simulink model "hw3_scattering_teleop_FP_nodamp"  (R2023b)
settings: Solver=ode45  StartTime=0.0  StopTime=10.0  FixedStep=0.001  RelTol=1e-3
values from neighbouring files (symbols this model uses):
  A = 1    [Copy_of_hw1_four_channel_bilateral_teleoperation_params.m]    (also in hw1_four_channel_bilateral_teleoperation_params.m; hw2_2_3_channel_bilateral_teleoperation_params.m; hw3_scattering_teleop_FP_params.m = 1.5; hw3_scattering_teleop_PP_params.m)
  Ak = [1 Ts ... (first row only)    [hw3_scattering_teleop_FP_params.m]    (also in hw3_scattering_teleop_PP_params.m; hw4_tank_FP_params.m; hw4_tank_PP_params.m; no_noise_hw4_tank_PP_params.m)
  B = [Ts^2/2; Ts]    [hw3_scattering_teleop_FP_params.m]    (also in hw3_scattering_teleop_PP_params.m; hw4_tank_FP_params.m; hw4_tank_PP_params.m; no_noise_hw4_tank_PP_params.m)
  b = 1    [hw3_scattering_teleop_FP_params.m]    (also in hw3_scattering_teleop_PP_params.m)
  Be = 100    [Copy_of_hw1_four_channel_bilateral_teleoperation_params.m]    (also in hw1_four_channel_bilateral_teleoperation_params.m; hw2_2_3_channel_bilateral_teleoperation_params.m; hw3_scattering_teleop_FP_params.m; hw3_scattering_teleop_PP_params.m)
  Bh = 1    [Copy_of_hw1_four_channel_bilateral_teleoperation_params.m]    (also in hw1_four_channel_bilateral_teleoperation_params.m; hw2_2_3_channel_bilateral_teleoperation_params.m; hw3_scattering_teleop_FP_params.m; hw3_scattering_teleop_PP_params.m)
  Bs = 4*Bm    (= 64)    [Copy_of_hw1_four_channel_bilateral_teleoperation_params.m]    (also in hw1_four_channel_bilateral_teleoperation_params.m; hw2_2_3_channel_bilateral_teleoperation_params.m; hw3_scattering_teleop_FP_params.m; hw3_scattering_teleop_PP_params.m)
  C = [1 0]    [hw3_scattering_teleop_FP_params.m]    (also in hw3_scattering_teleop_PP_params.m; hw4_tank_FP_params.m; hw4_tank_PP_params.m; no_noise_hw4_tank_PP_params.m)
  d = 1    [hw2_2_3_channel_bilateral_teleoperation_params.m]    (also in hw3_scattering_teleop_FP_params.m = 10; hw3_scattering_teleop_PP_params.m = 10; hw4_tank_FP_params.m = 10; hw4_tank_PP_params.m = 10)
  Dh = 20*0.8    (= 16)    [Copy_of_hw1_four_channel_bilateral_teleoperation_params.m]    (also in hw1_four_channel_bilateral_teleoperation_params.m; hw2_2_3_channel_bilateral_teleoperation_params.m; hw3_scattering_teleop_FP_params.m; hw3_scattering_teleop_PP_params.m)
  Dm = 5    [Copy_of_hw1_four_channel_bilateral_teleoperation_params.m]    (also in hw1_four_channel_bilateral_teleoperation_params.m; hw2_2_3_channel_bilateral_teleoperation_params.m; hw3_scattering_teleop_FP_params.m; hw3_scattering_teleop_PP_params.m = 0)
  Ds = 10    [Copy_of_hw1_four_channel_bilateral_teleoperation_params.m]    (also in hw1_four_channel_bilateral_teleoperation_params.m; hw2_2_3_channel_bilateral_teleoperation_params.m; hw3_scattering_teleop_FP_params.m = 0; hw3_scattering_teleop_PP_params.m = 0)
  Fc = 1    [Copy_of_hw1_four_channel_bilateral_teleoperation_params.m]    (also in hw1_four_channel_bilateral_teleoperation_params.m; hw2_2_3_channel_bilateral_teleoperation_params.m; hw3_scattering_teleop_FP_params.m; hw3_scattering_teleop_PP_params.m)
  Fip = 5    [hw3_scattering_teleop_FP_params.m]    (also in hw3_scattering_teleop_PP_params.m)
  Flp = 0.5    [Copy_of_hw1_four_channel_bilateral_teleoperation_params.m]    (also in hw1_four_channel_bilateral_teleoperation_params.m; hw2_2_3_channel_bilateral_teleoperation_params.m; hw3_scattering_teleop_FP_params.m = 0.01; hw3_scattering_teleop_PP_params.m = 0.01)
  Flp1 = 0.5    [hw3_scattering_teleop_FP_params.m]    (also in hw3_scattering_teleop_PP_params.m; hw4_tank_FP_params.m; hw4_tank_PP_params.m; no_noise_hw4_tank_PP_params.m)
  Jh = 1    [Copy_of_hw1_four_channel_bilateral_teleoperation_params.m]    (also in hw1_four_channel_bilateral_teleoperation_params.m; hw2_2_3_channel_bilateral_teleoperation_params.m; hw3_scattering_teleop_FP_params.m; hw3_scattering_teleop_PP_params.m)
  Ke = 200    [Copy_of_hw1_four_channel_bilateral_teleoperation_params.m]    (also in hw1_four_channel_bilateral_teleoperation_params.m; hw2_2_3_channel_bilateral_teleoperation_params.m; hw3_scattering_teleop_FP_params.m; hw3_scattering_teleop_PP_params.m)
  Kh = 0    [hw3_scattering_teleop_FP_params.m]    (also in hw3_scattering_teleop_PP_params.m; hw4_tank_FP_params.m; hw4_tank_PP_params.m; no_noise_hw4_tank_PP_params.m)
  Ks = 4*Km    (= 40)    [Copy_of_hw1_four_channel_bilateral_teleoperation_params.m]    (also in hw1_four_channel_bilateral_teleoperation_params.m; hw2_2_3_channel_bilateral_teleoperation_params.m; hw3_scattering_teleop_FP_params.m; hw3_scattering_teleop_PP_params.m)
  Mm = 0.5    [Copy_of_hw1_four_channel_bilateral_teleoperation_params.m]    (also in hw1_four_channel_bilateral_teleoperation_params.m; hw2_2_3_channel_bilateral_teleoperation_params.m; hw3_scattering_teleop_FP_params.m; hw3_scattering_teleop_PP_params.m)
  Ms = 2    [Copy_of_hw1_four_channel_bilateral_teleoperation_params.m]    (also in hw1_four_channel_bilateral_teleoperation_params.m; hw2_2_3_channel_bilateral_teleoperation_params.m; hw3_scattering_teleop_FP_params.m; hw3_scattering_teleop_PP_params.m)
  noise = 0.001    [hw3_scattering_teleop_FP_params.m]    (also in hw3_scattering_teleop_PP_params.m; hw4_tank_FP_params.m = 0.0001; hw4_tank_PP_params.m; no_noise_hw4_tank_PP_params.m)
  Ph = 10*1    (= 10)    [Copy_of_hw1_four_channel_bilateral_teleoperation_params.m]    (also in hw1_four_channel_bilateral_teleoperation_params.m; hw2_2_3_channel_bilateral_teleoperation_params.m; hw3_scattering_teleop_FP_params.m; hw3_scattering_teleop_PP_params.m)
  R = 1    [hw3_scattering_teleop_FP_params.m]    (also in hw3_scattering_teleop_PP_params.m; hw4_tank_FP_params.m; hw4_tank_PP_params.m; no_noise_hw4_tank_PP_params.m)
  Ts = 0.001    [hw3_scattering_teleop_FP_params.m]    (also in hw3_scattering_teleop_PP_params.m; hw4_tank_FP_params.m; hw4_tank_PP_params.m; no_noise_hw4_tank_PP_params.m)
  x0 = [0 0]    [hw3_scattering_teleop_FP_params.m]    (also in hw3_scattering_teleop_PP_params.m; hw4_tank_FP_params.m; hw4_tank_PP_params.m; no_noise_hw4_tank_PP_params.m)
  xe = 5    [Copy_of_hw1_four_channel_bilateral_teleoperation_params.m]    (also in hw1_four_channel_bilateral_teleoperation_params.m = 0.8; hw2_2_3_channel_bilateral_teleoperation_params.m = 2; hw3_scattering_teleop_FP_params.m = 0.8; hw3_scattering_teleop_PP_params.m = 2)
undefined symbols (not defined in the file or in its folder): DiscIntNeverNeededParam, Discrete, Time
libraries: simulink x3, ctrlSharedLib x2, cstblocks x1
settings Model: Creator=86180  LastModifiedBy=86180

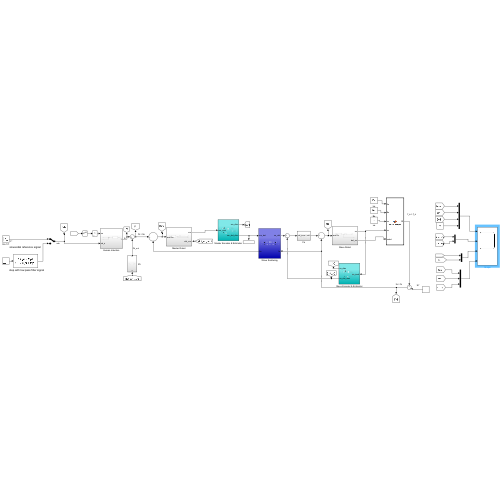
[thumbnail: Simulink's stored preview of the top-level diagram]
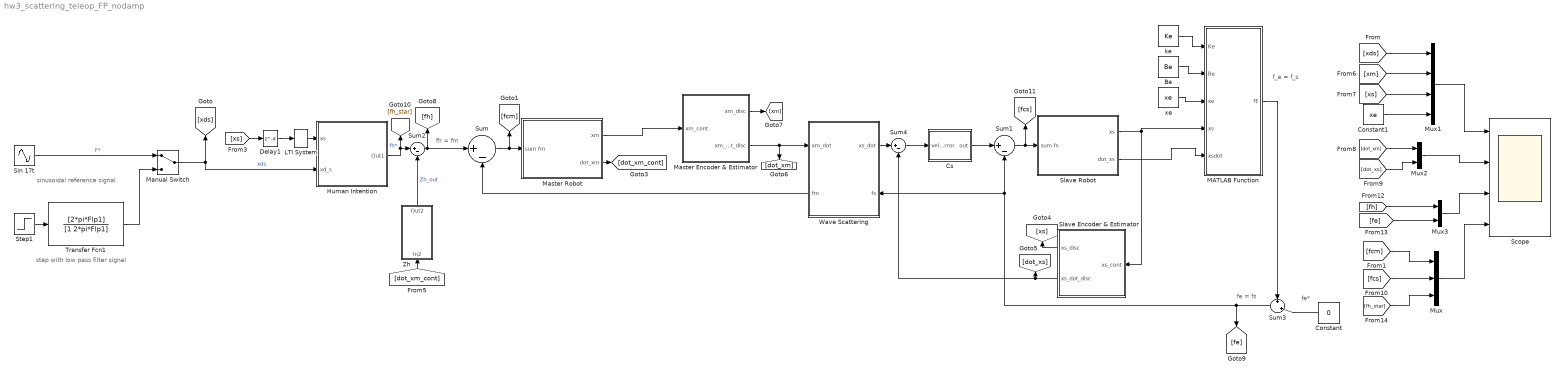
== system hw3_scattering_teleop_FP_nodamp ==
  note: f_e = f_s
  note: fe*
  note: fe = fs
  note: fh = fm
  note: sinusoidal reference signal
  note: step with low pass filter signal
  Be : Constant  Value=Be
  Constant : Constant  Value=0
  Constant1 : Constant  Value=xe
  Cs : Subsystem
  Delay1 : Delay  DelayLength=d
  Human Intention : Subsystem
  LTI System : cstblocks/LTI System  sys=1  IC=[]  PadeOrder=0
  MATLAB Function : MATLAB Function  TreatAsAtomicUnit=on
  Manual Switch : ManualSwitch
  Master Encoder & Estimator : Subsystem
  Master Robot : Subsystem
  Mux : Mux  Inputs=3
  Mux1 : Mux
  Mux2 : Mux  Inputs=2
  Mux3 : Mux  Inputs=2
  Scope : Scope  NumInputPorts=4
  Sin 17t : Sin  Amplitude=A  Frequency=2*pi*Fc  SampleTime=0
  Slave Encoder & Estimator : Subsystem
  Slave Robot : Subsystem
  Step1 : Step  Time=0.5  After=A  SampleTime=0
  Sum{,1..2,4} (4 alike) : Sum  Inputs=|+-
  Sum3 : Sum  Inputs=+|+|
  Transfer Fcn1 : TransferFcn  Numerator=[2*pi*Flp1]  Denominator=[1 2*pi*Flp1]
  Wave Scattering : Subsystem
      settings: PortSchema="{\"entries\":[{\"content\":{\"sides\":[{\"content\":{\"connectorIds\":[\"In1\",\"Out2\"]},\"type\":\"ConnectorPlacement.EquallySpacedRectSide\",\"uuid\":\"0c50569d-963b-48ab-a577-26f0d9876433\"},{\"content\":{\"connectorIds\":[\"Out1\",\"In2\"],\"side\":\"RIGHT\"},\"type\":\"ConnectorPlacement.EquallySpacedRectSide\",\"uuid\":\"037c0148-99ff-4004-98e0-dcfb6e9384bd\"},{\"content\":{\"side\":\"TOP\"},\"type\":\"ConnectorPlacement.EquallySpacedRectSide\",\"uuid\":\"ad6d8fee-2812-437e-9537-eb4f2a26ae7c\"}]},\"type\":\"ConnectorPlacement.EquallySpacedConnector\",\"uuid\":\"8c48c0e6-767c-4561-83e1-39f24f1e71e4\"}],\"packageUris\":[\"http://schema.mathworks.com/mf0/Connector/R2020b\"],\"version\":\"1.0\"}"
  Zh : Subsystem
  ke : Constant  Value=Ke
  xe : Constant  Value=xe
  wires:
  Manual Switch/1 -> Human Intention/2(xd_s), [xds]  "xds"
  Zh/1(Out2) -> Sum2/2  "Zh_out"
  Transfer Fcn1/1 -> Manual Switch/2
  Human Intention/1(Out1) -> [fh_star], Sum2/1  "fh*"
  Sin 17t/1 -> Manual Switch/1  "F*"
  Step1/1 -> Transfer Fcn1/1
  ke/1 -> MATLAB Function/1(Ke)
  xe/1 -> MATLAB Function/3(xe)
  Slave Robot/1(xs) -> MATLAB Function/4(xs), Slave Encoder & Estimator/1(xs_cont)
  MATLAB Function/1(fE) -> Sum3/1
  Be/1 -> MATLAB Function/2(Be)
  Sum2/1 -> Sum/1, [fh]
  Slave Robot/2(dot_xs) -> MATLAB Function/5(xsdot)
  Sum3/1 -> Sum1/2, Wave Scattering/2(fs), [fe]
  Constant/1 -> Sum3/2
  [xds] -> Mux1/1
  Sum/1 -> [fcm], Master Robot/1(sum fm)
  [dot_xm_cont] -> Zh/1(In2)
  [xm] -> Mux1/2
  [xs] -> Mux1/3
  [dot_xm] -> Mux2/1
  Sum1/1 -> [fcs], Slave Robot/1(sum fs)
  [fh] -> Mux3/1
  [fe] -> Mux3/2
  [fh_star] -> Mux/3
  [fcs] -> Mux/2
  [fcm] -> Mux/1
  Constant1/1 -> Mux1/4
  [dot_xs] -> Mux2/2
  Mux1/1 -> Scope/1
  Mux2/1 -> Scope/2
  Mux3/1 -> Scope/3
  Mux/1 -> Scope/4
  [xs] -> Delay1/1
  Master Robot/1(xm) -> Master Encoder & Estimator/1(xm_cont)
  Master Encoder & Estimator/1(xm_disc) -> [xm]
  Master Encoder & Estimator/2(xm_dot_disc) -> [dot_xm], Wave Scattering/1(xm_dot)
  Wave Scattering/1(xs_dot) -> Sum4/1
  Wave Scattering/2(fm) -> Sum/2
  Sum4/1 -> Cs/1(vel_error)
  Cs/1(out) -> Sum1/1
  Slave Encoder & Estimator/2(xs_dot_disc) -> [dot_xs], Sum4/2
  Slave Encoder & Estimator/1(xs_disc) -> [xs]
  Delay1/1 -> LTI System/1
  LTI System/1 -> Human Intention/1(xs)
  Master Robot/2(dot_xm) -> [dot_xm_cont]

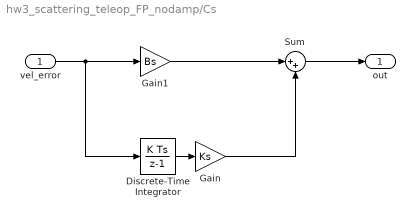
== system hw3_scattering_teleop_FP_nodamp/Cs ==
  vel_error : Inport
  Discrete-Time Integrator : DiscreteIntegrator  SampleTime=-1  ICPrevOutput=DiscIntNeverNeededParam  ICPrevScaledInput=DiscIntNeverNeededParam
  Gain : Gain  Gain=Ks
  Gain1 : Gain  Gain=Bs
  Sum : Sum  Inputs=|++
  out : Outport
  wires:
  Gain/1 -> Sum/2
  vel_error/1 -> Discrete-Time Integrator/1, Gain1/1
  Discrete-Time Integrator/1 -> Gain/1
  Sum/1 -> out/1
  Gain1/1 -> Sum/1

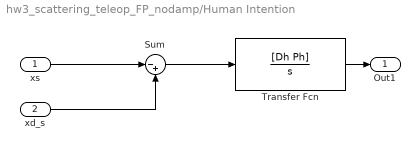
== system hw3_scattering_teleop_FP_nodamp/Human Intention ==
  xs : Inport
  xd_s : Inport  Port=2
  Sum : Sum  Inputs=|-+
  Transfer Fcn : TransferFcn  Numerator=[Dh Ph]  Denominator=[1 0]
  Out1 : Outport
  wires:
  Sum/1 -> Transfer Fcn/1
  xd_s/1 -> Sum/2
  xs/1 -> Sum/1
  Transfer Fcn/1 -> Out1/1

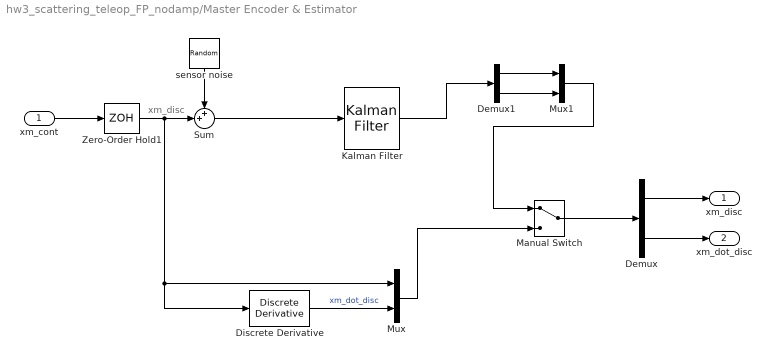
== system hw3_scattering_teleop_FP_nodamp/Master Encoder & Estimator ==
  note: xm_disc
  xm_cont : Inport
  Demux : Demux  Outputs=2
  Demux1 : Demux  Outputs=2
  Discrete Derivative : simulink/Discrete/Discrete Derivative  gainval=1.0  ICPrevScaledInput=0.0  OutMin=[]  OutMax=[]  OutDataType=fixdt(1, 16)  OutScaling=2^-10  DoSatur=off
  Kalman Filter : ctrlSharedLib/Kalman Filter  TimeDomain=Discrete-Time  UseCurrentEstimator=on  ModelSource=Individual A, B, C, D matrices  ModelSourceVariable=ss(0.95,1,1,0,1)  A=Ak  B=B  C=C  D=0  NumberOfStates=2  NumberOfInputs=1  NumberOfOutputs=1  InitialEstimateSource=Dialog  X0=x0  P0=10  UseK=off  UseGH=off  NumberOfProcessNoiseInputs=1  G=1  TimeInvariantG=on  H=0  TimeInvariantH=on  Q=Q_m  TimeInvariantQ=on  R=R  TimeInvariantR=on  N=0  TimeInvariantN=on  AddInputPort=off  AddEnablePort=off  OutputEstimatedY=off  OutputP=off  Ts=Ts
  Manual Switch : ManualSwitch
  Mux : Mux  Inputs=2
  Mux1 : Mux  Inputs=2
  Sum : Sum  Inputs=++|
  Zero-Order Hold1 : ZeroOrderHold  SampleTime=Ts
  sensor noise : RandomNumber  Variance=noise  SampleTime=Ts
  xm_disc : Outport
  xm_dot_disc : Outport  Port=2
  wires:
  Demux/2 -> xm_dot_disc/1
  Discrete Derivative/1 -> Mux/2  "xm_dot_disc"
  Manual Switch/1 -> Demux/1
  Zero-Order Hold1/1 -> Mux/1, Discrete Derivative/1, Sum/2
  xm_cont/1 -> Zero-Order Hold1/1
  Demux/1 -> xm_disc/1
  sensor noise/1 -> Sum/1
  Mux/1 -> Manual Switch/2
  Mux1/1 -> Manual Switch/1
  Sum/1 -> Kalman Filter/1
  Kalman Filter/1 -> Demux1/1
  Demux1/1 -> Mux1/1
  Demux1/2 -> Mux1/2

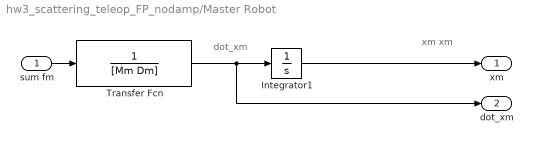
== system hw3_scattering_teleop_FP_nodamp/Master Robot ==
  note: dot_xm
  note: xm
      | xm
  sum fm : Inport
  Integrator1 : Integrator
  Transfer Fcn : TransferFcn  Denominator=[Mm Dm]
  xm : Outport
  dot_xm : Outport  Port=2
  wires:
  Integrator1/1 -> xm/1
  Transfer Fcn/1 -> dot_xm/1, Integrator1/1
  sum fm/1 -> Transfer Fcn/1

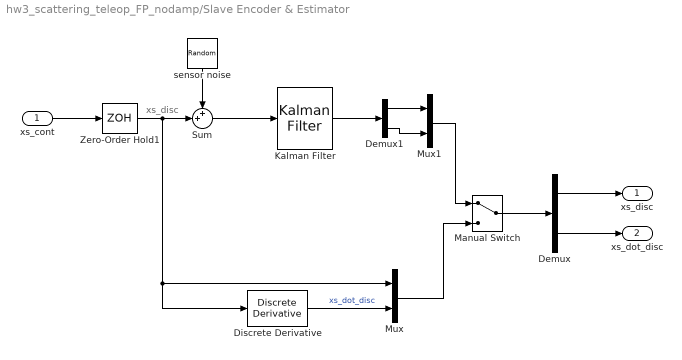
== system hw3_scattering_teleop_FP_nodamp/Slave Encoder & Estimator ==
  note: xs_disc
  xs_cont : Inport
  Demux : Demux  Outputs=2
  Demux1 : Demux  Outputs=2
  Discrete Derivative : simulink/Discrete/Discrete Derivative  gainval=1.0  ICPrevScaledInput=0.0  OutMin=[]  OutMax=[]  OutDataType=fixdt(1, 16)  OutScaling=2^-10  DoSatur=off
  Kalman Filter : ctrlSharedLib/Kalman Filter  TimeDomain=Discrete-Time  UseCurrentEstimator=on  ModelSource=Individual A, B, C, D matrices  ModelSourceVariable=ss(0.95,1,1,0,1)  A=Ak  B=B  C=C  D=0  NumberOfStates=2  NumberOfInputs=1  NumberOfOutputs=1  InitialEstimateSource=Dialog  X0=0  P0=10  UseK=off  UseGH=off  NumberOfProcessNoiseInputs=1  G=1  TimeInvariantG=on  H=0  TimeInvariantH=on  Q=Q_m  TimeInvariantQ=on  R=R  TimeInvariantR=on  N=0  TimeInvariantN=on  AddInputPort=off  AddEnablePort=off  OutputEstimatedY=off  OutputP=off  Ts=Ts
  Manual Switch : ManualSwitch
  Mux : Mux  Inputs=2
  Mux1 : Mux  Inputs=2
  Sum : Sum  Inputs=++|
  Zero-Order Hold1 : ZeroOrderHold  SampleTime=Ts
  sensor noise : RandomNumber  Variance=noise  SampleTime=Ts
  xs_disc : Outport
  xs_dot_disc : Outport  Port=2
  wires:
  Demux/2 -> xs_dot_disc/1
  Discrete Derivative/1 -> Mux/2  "xs_dot_disc"
  Manual Switch/1 -> Demux/1
  Zero-Order Hold1/1 -> Mux/1, Discrete Derivative/1, Sum/2
  xs_cont/1 -> Zero-Order Hold1/1
  Demux/1 -> xs_disc/1
  sensor noise/1 -> Sum/1
  Mux/1 -> Manual Switch/2
  Sum/1 -> Kalman Filter/1
  Mux1/1 -> Manual Switch/1
  Kalman Filter/1 -> Demux1/1
  Demux1/1 -> Mux1/1
  Demux1/2 -> Mux1/2

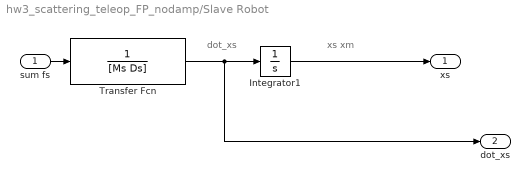
== system hw3_scattering_teleop_FP_nodamp/Slave Robot ==
  note: dot_xs
  note: xs
      | xm
  sum fs : Inport
  Integrator1 : Integrator
  Transfer Fcn : TransferFcn  Denominator=[Ms Ds]
  xs : Outport
  dot_xs : Outport  Port=2
  wires:
  Integrator1/1 -> xs/1
  Transfer Fcn/1 -> dot_xs/1, Integrator1/1
  sum fs/1 -> Transfer Fcn/1

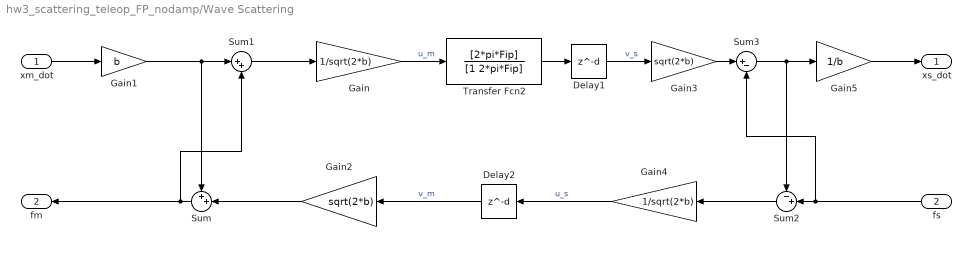
== system hw3_scattering_teleop_FP_nodamp/Wave Scattering ==
  xm_dot : Inport
  fs : Inport  Port=2
  Delay1 : Delay  DelayLength=d  SampleTime=Ts
  Delay2 : Delay  DelayLength=d  SampleTime=Ts
  Gain : Gain  Gain=1/sqrt(2*b)
  Gain1 : Gain  Gain=b
  Gain2 : Gain  Gain=sqrt(2*b)
  Gain3 : Gain  Gain=sqrt(2*b)
  Gain4 : Gain  Gain=1/sqrt(2*b)
  Gain5 : Gain  Gain=1/b
  Sum : Sum  Inputs=++|
  Sum1 : Sum  Inputs=|++
  Sum2 : Sum  Inputs=-+|
  Sum3 : Sum  Inputs=|+-
  Transfer Fcn2 : TransferFcn  Numerator=[2*pi*Fip]  Denominator=[1 2*pi*Fip]
  xs_dot : Outport
  fm : Outport  Port=2
  wires:
  Gain3/1 -> Sum3/1
  Gain5/1 -> xs_dot/1
  Sum/1 -> fm/1, Sum1/2
  Transfer Fcn2/1 -> Delay1/1
  Delay2/1 -> Gain2/1  "v_m"
  xm_dot/1 -> Gain1/1
  Sum3/1 -> Sum2/1, Gain5/1
  Delay1/1 -> Gain3/1  "v_s"
  fs/1 -> Sum3/2, Sum2/2
  Gain4/1 -> Delay2/1  "u_s"
  Gain2/1 -> Sum/2
  Gain1/1 -> Sum1/1, Sum/1
  Gain/1 -> Transfer Fcn2/1  "u_m"
  Sum1/1 -> Gain/1
  Sum2/1 -> Gain4/1

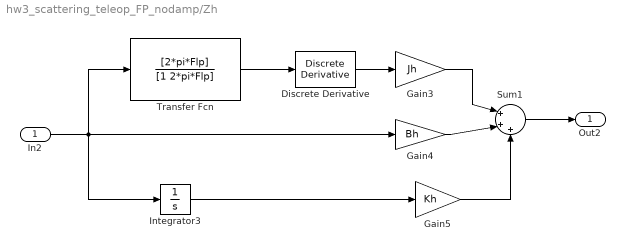
== system hw3_scattering_teleop_FP_nodamp/Zh ==
  In2 : Inport
  Discrete Derivative : simulink/Discrete/Discrete Derivative  gainval=1.0  ICPrevScaledInput=0.0  OutMin=[]  OutMax=[]  OutDataType=fixdt(1, 16)  OutScaling=2^-10  DoSatur=off
  Gain3 : Gain  Gain=Jh
  Gain4 : Gain  Gain=Bh
  Gain5 : Gain  Gain=Kh
  Integrator3 : Integrator
  Sum1 : Sum  Inputs=|+++
  Transfer Fcn : TransferFcn  Numerator=[2*pi*Flp]  Denominator=[1 2*pi*Flp]
  Out2 : Outport
  wires:
  Gain3/1 -> Sum1/1
  In2/1 -> Transfer Fcn/1, Integrator3/1, Gain4/1
  Gain5/1 -> Sum1/3
  Gain4/1 -> Sum1/2
  Integrator3/1 -> Gain5/1
  Transfer Fcn/1 -> Discrete Derivative/1
  Discrete Derivative/1 -> Gain3/1
  Sum1/1 -> Out2/1

== matlab function hw3_scattering_teleop_FP_nodamp/MATLAB Function ==
  data: Ke input; fE output; Be input; xe input; xs input; xsdot input
function fE = environment(Ke, Be, xe, xs, xsdot)
    if xs > xe
        fE = Ke * (xs - xe) + Be * xsdot; % Plot both contributions Ke and Be
    else
        fE = 0;
    end
end
